simulink model "CC_CV_Charger"  (Simulink 10.0)
settings: Solver=ode23tb  StartTime=0  StopTime=inf  RelTol=1e-4  EnableMultiTasking=on
undefined symbols (not defined in the file): f, Ion, Lithium
libraries: powerlib x12, simulink x3, electricdrivelib x1
settings Model: Creator=LMPhuong  LastModifiedBy=bhisma
settings SolverCC: ZeroCrossControl=DisableAll
settings DataIOCC: LimitDataPoints=on  SignalLoggingSaveFormat=ModelDataLogs  SignalLoggingName=sigsOut
settings OptimizationCC: ExpressionDepthLimit=2147483647  InitFltsAndDblsToZero=on
settings DebuggingCC: SaveWithParameterizedLinksMsg=none  SignalResolutionControl=TryResolveAllWithWarning  MultiTaskDSMMsg=warning  MultiTaskCondExecSysMsg=none  FcnCallInpInsideContextMsg=warning  StateNameClashWarn=warning
settings HardwareCC: TargetBitPerLong=64  TargetBitPerPointer=64  TargetBitPerSizeT=64  TargetBitPerPtrDiffT=64  TargetLongLongMode=on  TargetIntDivRoundTo=Zero  TargetEndianess=LittleEndian  TargetWordSize=64  TargetHWDeviceType=MATLAB Host  ProdEqTarget=off
settings GRTTargetCC: TargetFcnLib=ansi_tfl_tmw.mat  GeneratePreprocessorConditionals=Disable all
settings ConfigComp: CovExternalEMLEnable=off
settings SimscapeCC: SimscapeNormalizeSystem=off

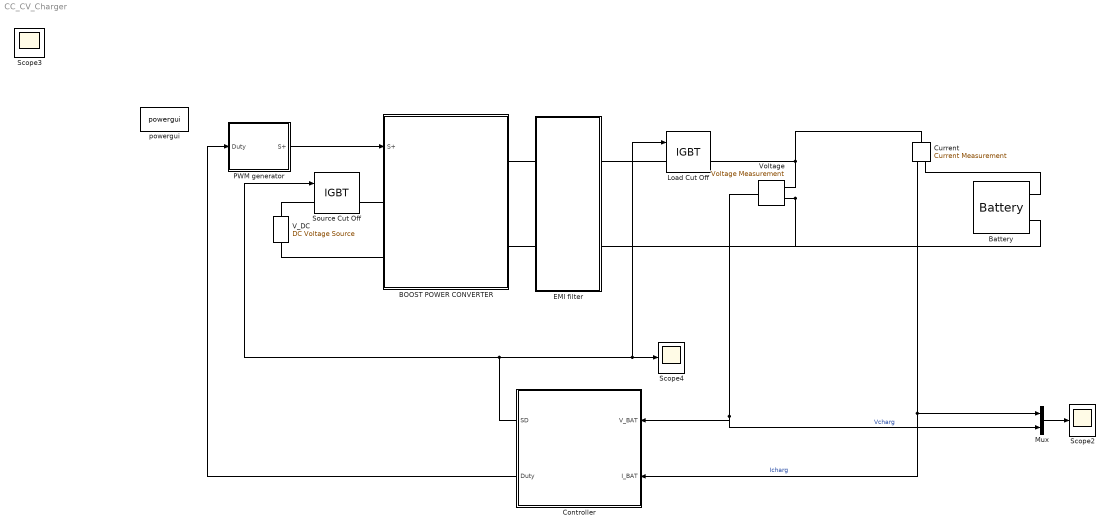
== system CC_CV_Charger ==
  BOOST POWER CONVERTER : Subsystem
  Battery : electricdrivelib/Extra Sources/Battery  BatType=Lithium-Ion  ShowDetailedParameters=off  NomV=48  NomQ=100  SOC=99.7  PresetModel=off  MaxQ=100  FullV=58.4  Dis_rate=0  R=0.0048  Normal_OP=90.4348  expZone="[51.8585      4.91304]"  Dis_Char=off  current=[20 100]  Units=Ampere-hour  Batt_Tr=30
      link override Series RLC Branch: Resistance=0.013
      settings: SourceProductName=Simscape Electrical
  Controller : Subsystem
  Current : powerlib/Measurements/Current Measurement  PhasorSimulation=off  OutputType=Complex  PSBequivalent=0
      settings: SourceProductName=Simscape Electrical
  EMI filter : Subsystem
  Load Cut Off : powerlib/Power Electronics/IGBT  Ron=0.018  Lon=0  Vf=0.3  Tf=0  Tt=0  IC=0  Rs=1e5  Cs=inf  Measurements=on
      settings: SourceProductName=Simscape Electrical
  Mux : Mux  Inputs=2
  PWM generator : Subsystem
  Scope2 : Scope
  Scope4 : Scope
  Source Cut Off : powerlib/Power Electronics/IGBT  Ron=0.00001  Lon=0  Vf=0.3  Tf=0  Tt=0  IC=0  Rs=1e5  Cs=inf  Measurements=on
      settings: SourceProductName=Simscape Electrical
  V_DC : powerlib/Electrical Sources/DC Voltage Source  Amplitude=32  Measurements=Voltage
      settings: SourceProductName=Simscape Electrical
  Voltage : powerlib/Measurements/Voltage Measurement  PhasorSimulation=off  OutputType=Complex  PSBequivalent=0
      settings: SourceProductName=Simscape Electrical
  powergui : powerlib/powergui  SimulationMode=Discrete  SolverType=Tustin  SampleTime=1e-6  frequency=60  SPID=off  DisableSnubberDevices=off  DisableRonSwitches=off  DisableVfSwitches=off  SwTol=0  Interpol=off  DisplayEquations=off  FunctionMessages=off  frequencyindice=0  Pbase=100e6  ErrMax=1e-4  Iterations=50  UnitsV=kV  UnitsW=MW  echomessages=off  HookPort=off  EnableUseOfTLC=off  x0status=blocks  RestoreLinks=warning  ResistiveCurrentMeasurement=off  Frange=[0:2:500]  Ylog=off  Xlog=on  ShowGrid=off  save=off  variable=ZData  structure=ScopeData  ZoomFFT=off  StartTime=0.04  cycles=2  DisplayStyle=1  fundamental=1000  FreqAxis=off  MaxFrequency=50000  frequencyindicesteady=1  RmsSteady=1  display=off  Ts=0  methode=off
      settings: SourceProductName=Simscape Electrical
  Scope3 : Scope
  wires:
  Current/1 -> Controller/2(I_BAT), Mux/1  "Icharg"
  Voltage/1 -> Controller/1(V_BAT), Mux/2  "Vcharg"
  PWM generator/1(S+) -> BOOST POWER CONVERTER/1(S+)
  Controller/1(SD) -> Scope4/1, Load Cut Off/1, Source Cut Off/1
  Controller/2(Duty) -> PWM generator/1(Duty)
  Mux/1 -> Scope2/1
  connections:
  Current/RConn1 -- Battery/LConn1
  BOOST POWER CONVERTER/RConn1 -- EMI filter/LConn1
  EMI filter/LConn2 -- BOOST POWER CONVERTER/RConn2
  BOOST POWER CONVERTER/LConn2 -- V_DC/LConn1
  Load Cut Off/RConn1 -- Voltage/LConn1 -- Current/LConn1
  Voltage/LConn2 -- Battery/LConn2 -- EMI filter/RConn2
  Load Cut Off/LConn1 -- EMI filter/RConn1
  Source Cut Off/RConn1 -- BOOST POWER CONVERTER/LConn1
  Source Cut Off/LConn1 -- V_DC/RConn1

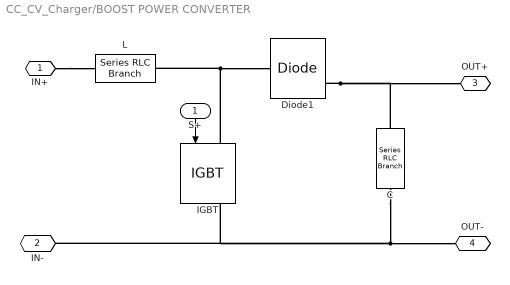
== system CC_CV_Charger/BOOST POWER CONVERTER ==
  S+ : Inport
  " C" : powerlib/Elements/Series RLC Branch  LConnTagsString=__new0  RConnTagsString=__new0  BranchType=C  Resistance=5  Inductance=0.05  SetiL0=off  InitialCurrent=0  Capacitance=100e-6  Setx0=on  InitialVoltage=0  Measurements=Branch voltage and current
      settings: SourceProductName=Simscape Electrical
  " L" : powerlib/Elements/Series RLC Branch  LConnTagsString=__new0  RConnTagsString=__new0  BranchType=L  Resistance=5  Inductance=10e-6  SetiL0=on  InitialCurrent=0  Capacitance=1.0  Setx0=off  InitialVoltage=0  Measurements=Branch voltage and current
      settings: SourceProductName=Simscape Electrical
  Diode1 : powerlib/Power Electronics/Diode  Ron=0.000001  Lon=0  Vf=0.8  IC=0  UseSnubber=off  Rs=1e4  Cs=1e-4  Measurements=on
      settings: SourceProductName=Simscape Electrical
  IGBT : powerlib/Power Electronics/IGBT  Ron=0.018  Lon=0  Vf=1  Tf=0  Tt=0  IC=0  Rs=1e5  Cs=inf  Measurements=on
      settings: SourceProductName=Simscape Electrical
  IN+ : PMIOPort  Side=Left
  IN- : PMIOPort  Port=2  Side=Left
  OUT+ : PMIOPort  Port=3  Side=Right
  OUT- : PMIOPort  Port=4  Side=Right
  wires:
  S+/1 -> IGBT/1
  connections:
  Diode1/RConn1 -- OUT+/RConn1 -- " C"/LConn1
  IGBT/RConn1 -- IN-/RConn1 -- OUT-/RConn1 -- " C"/RConn1
  IGBT/LConn1 -- " L"/RConn1 -- Diode1/LConn1
  IN+/RConn1 -- " L"/LConn1

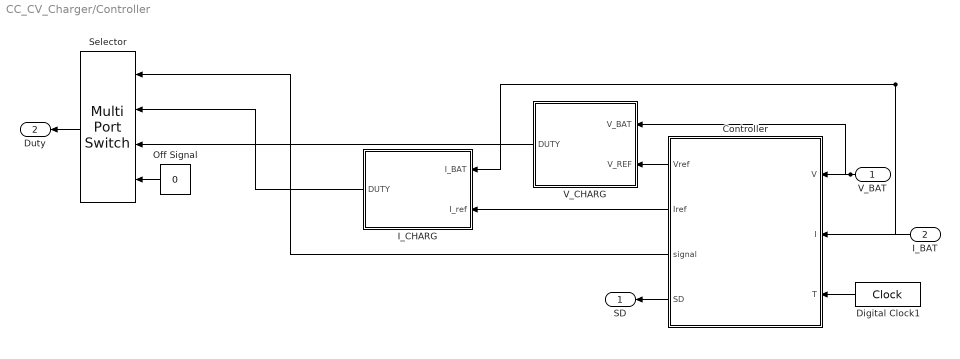
== system CC_CV_Charger/Controller ==
  V_BAT : Inport
  I_BAT : Inport  Port=2
  Controller : MATLAB Function  TreatAsAtomicUnit=on
  Digital Clock1 : DigitalClock  SampleTime=0.001
  I_CHARG : Subsystem
  Off Signal : Constant  Value=0
  Selector : MultiPortSwitch  DiagnosticForDefault=None
  V_CHARG : Subsystem
  SD : Outport
  Duty : Outport  Port=2
  wires:
  Controller/2(Iref) -> I_CHARG/2(I_ref)
  Digital Clock1/1 -> Controller/3(T)
  I_CHARG/1(DUTY) -> Selector/2
  Off Signal/1 -> Selector/4
  Controller/3(signal) -> Selector/1
  V_CHARG/1(DUTY) -> Selector/3
  I_BAT/1 -> I_CHARG/1(I_BAT), Controller/2(I)
  Selector/1 -> Duty/1
  Controller/4(SD) -> SD/1
  V_BAT/1 -> V_CHARG/1(V_BAT), Controller/1(V)
  Controller/1(Vref) -> V_CHARG/2(V_REF)

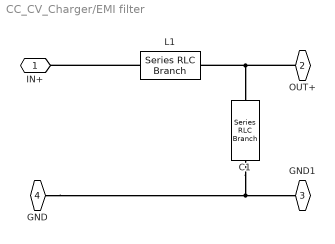
== system CC_CV_Charger/EMI filter ==
  " C1" : powerlib/Elements/Series RLC Branch  LConnTagsString=__new0  RConnTagsString=__new0  BranchType=C  Resistance=5  Inductance=0.05  SetiL0=off  InitialCurrent=0  Capacitance=1000e-6  Setx0=on  InitialVoltage=48  Measurements=Branch voltage and current
      settings: SourceProductName=Simscape Electrical
  " L1" : powerlib/Elements/Series RLC Branch  LConnTagsString=__new0  RConnTagsString=__new0  BranchType=L  Resistance=5  Inductance=0.005  SetiL0=on  InitialCurrent=0  Capacitance=1.0  Setx0=off  InitialVoltage=0  Measurements=Branch voltage and current
      settings: SourceProductName=Simscape Electrical
  IN+ : PMIOPort  Side=Left
  OUT+ : PMIOPort  Port=2  Side=Right
  GND1 : PMIOPort  Port=3  Side=Right
  GND : PMIOPort  Port=4  Side=Left
  connections:
  OUT+/RConn1 -- " L1"/RConn1 -- " C1"/LConn1
  " L1"/LConn1 -- IN+/RConn1
  GND/RConn1 -- GND1/RConn1 -- " C1"/RConn1

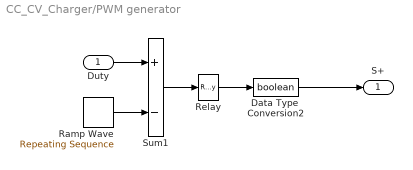
== system CC_CV_Charger/PWM generator ==
  Duty : Inport
  Data Type  Conversion2 : DataTypeConversion  OutDataTypeStr=boolean  SaturateOnIntegerOverflow=on  RndMeth=Zero
  Ramp Wave : simulink/Sources/Repeating Sequence  rep_seq_t=[0 1/20e3]  rep_seq_y=[0 1]
  Relay : Relay
  Sum1 : Sum  Inputs=+-  SaturateOnIntegerOverflow=on  InputSameDT=on  OutDataTypeStr=Inherit: Same as first input
  S+ : Outport
  wires:
  Data Type  Conversion2/1 -> S+/1
  Relay/1 -> Data Type  Conversion2/1
  Sum1/1 -> Relay/1
  Ramp Wave/1 -> Sum1/2
  Duty/1 -> Sum1/1

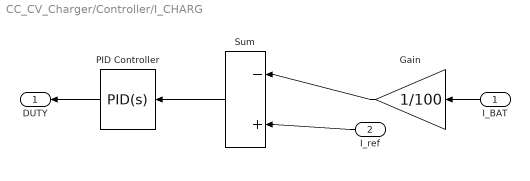
== system CC_CV_Charger/Controller/I_CHARG ==
  I_BAT : Inport
  I_ref : Inport  Port=2
  Gain : Gain  Gain=1/100
  PID Controller : simulink/Continuous/PID Controller  Controller=PID  TimeDomain=Continuous-time  SampleTime=1/f  IntegratorMethod=Forward Euler  FilterMethod=Forward Euler  Form=Parallel  P=0.75  I=50  D=3*2.7e-06  N=100  InitialConditionSource=internal  InitialConditionForIntegrator=0  InitialConditionForFilter=0  ExternalReset=none  LimitOutput=on  UpperSaturationLimit=0.9  LowerSaturationLimit=0  LinearizeAsGain=off  AntiWindupMode=none  Kb=1  TrackingMode=off  Kt=1  PParamMin=[]  PParamMax=[]  IParamMin=[]  IParamMax=[]  DParamMin=[]  DParamMax=[]  NParamMin=[]  NParamMax=[]  KbParamMin=[]  KbParamMax=[]  KtParamMin=[]  KtParamMax=[]  POutMin=[]  POutMax=[]  IOutMin=[]  IOutMax=[]  DOutMin=[]  DOutMax=[]  NOutMin=[]  NOutMax=[]  KbOutMin=[]  KbOutMax=[]  KtOutMin=[]  KtOutMax=[]  IntegratorOutMin=[]  IntegratorOutMax=[]  FilterOutMin=[]  FilterOutMax=[]  SumOutMin=[]  SumOutMax=[]  SumI1OutMin=[]  SumI1OutMax=[]  SumI2OutMin=[]  SumI2OutMax=[]  SumI3OutMin=[]  SumI3OutMax=[]  SumDOutMin=[]  SumDOutMax=[]  SaturationOutMin=[]  SaturationOutMax=[]  IntegratorContinuousStateAttributes=''  IntegratorStateMustResolveToSignalObject=off  IntegratorRTWStateStorageClass=Auto  FilterContinuousStateAttributes=''  FilterStateMustResolveToSignalObject=off  FilterRTWStateStorageClass=Auto
  Sum : Sum  Inputs=|-+
  DUTY : Outport
  wires:
  Sum/1 -> PID Controller/1
  I_BAT/1 -> Gain/1
  PID Controller/1 -> DUTY/1
  I_ref/1 -> Sum/2
  Gain/1 -> Sum/1

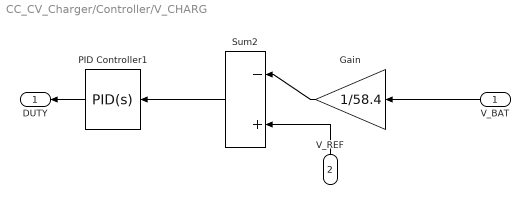
== system CC_CV_Charger/Controller/V_CHARG ==
  V_BAT : Inport
  V_REF : Inport  Port=2
  Gain : Gain  Gain=1/58.4
  PID Controller1 : simulink/Continuous/PID Controller  Controller=PID  TimeDomain=Continuous-time  SampleTime=1/f  IntegratorMethod=Forward Euler  FilterMethod=Forward Euler  Form=Parallel  P=0.65  I=150  D=2.7e-06  N=100  InitialConditionSource=internal  InitialConditionForIntegrator=0  InitialConditionForFilter=0  ExternalReset=none  LimitOutput=on  UpperSaturationLimit=0.9  LowerSaturationLimit=0  LinearizeAsGain=off  AntiWindupMode=none  Kb=1  TrackingMode=off  Kt=1  PParamMin=[]  PParamMax=[]  IParamMin=[]  IParamMax=[]  DParamMin=[]  DParamMax=[]  NParamMin=[]  NParamMax=[]  KbParamMin=[]  KbParamMax=[]  KtParamMin=[]  KtParamMax=[]  POutMin=[]  POutMax=[]  IOutMin=[]  IOutMax=[]  DOutMin=[]  DOutMax=[]  NOutMin=[]  NOutMax=[]  KbOutMin=[]  KbOutMax=[]  KtOutMin=[]  KtOutMax=[]  IntegratorOutMin=[]  IntegratorOutMax=[]  FilterOutMin=[]  FilterOutMax=[]  SumOutMin=[]  SumOutMax=[]  SumI1OutMin=[]  SumI1OutMax=[]  SumI2OutMin=[]  SumI2OutMax=[]  SumI3OutMin=[]  SumI3OutMax=[]  SumDOutMin=[]  SumDOutMax=[]  SaturationOutMin=[]  SaturationOutMax=[]  IntegratorContinuousStateAttributes=''  IntegratorStateMustResolveToSignalObject=off  IntegratorRTWStateStorageClass=Auto  FilterContinuousStateAttributes=''  FilterStateMustResolveToSignalObject=off  FilterRTWStateStorageClass=Auto
  Sum2 : Sum  Inputs=|-+
  DUTY : Outport
  wires:
  Sum2/1 -> PID Controller1/1
  V_REF/1 -> Sum2/2
  PID Controller1/1 -> DUTY/1
  V_BAT/1 -> Gain/1
  Gain/1 -> Sum2/1

== matlab function Controller/Controller ==
  data: Vref output double; Iref output double; V input double; I input double; T input double; signal output double; SD output double
function [Vref,Iref,signal,SD] = CHARGER(V,I,T)
persistent temp_i temp_v temp_signal temp_fault CC CV n ;
if isempty(temp_i)
    temp_i=0.2;
end
if isempty(temp_v)
    temp_v=0;
end
if isempty(temp_signal)
    temp_signal=1;
end
if isempty(temp_fault)
    temp_fault=1;
end
if isempty(CC)
    CC=1;
end
if isempty(CV)
    CV=0;
end
if isempty(n)
    n=0;
end
if (T>n*0.02) % sample time is 0.02s
    n=n+1;
    if CC
        if V<58.4    
            temp_i=1;
            temp_v=0;
            temp_signal=1;
        else
            CV=1;
        end
    end
    if CV
        if I>5.0
            temp_i=0;
            temp_v=1;
            temp_signal=2;
        else
            temp_fault=0;
        end
    end
end
signal=temp_signal;
SD=temp_fault;
Iref=temp_i;
Vref=temp_v;
end
